simulink model "Simscape_exercise3"  (R2015b)
settings: Solver=ode23t  SolverMode=SingleTasking  StartTime=0.0  StopTime=5  RelTol=1e-3
values from neighbouring files (symbols this model uses):
  Amplitude = 2    [Exercise_3.m]
  Freq = 2    [Exercise_3.m]
  Jm = 7.46/(1000*100^2)    (= 7.46e-07)    [Exercise_1.m]    (also in Exercise_3.m)
  Sine_wave = 1    [Exercise_3.m]
  voltage = 1    [Exercise_3.m]
libraries: fl_lib x10, nesl_utility x6, simulink x1, elec_lib x1
settings Model: Creator=diegogm  LastModifiedBy=sofianh
settings DataIOCC: SaveFormat=Array
settings OptimizationCC: BlockReduction=off  BooleanDataType=off
settings DebuggingCC: SaveWithParameterizedLinksMsg=none  UnderspecifiedInitializationDetection=Classic  MergeDetectMultiDrivingBlocksExec=none  SignalResolutionControl=TryResolveAllWithWarning
settings HardwareCC: ProdBitPerPointer=32  ProdLargestAtomicFloat=None  ProdIntDivRoundTo=Undefined  ProdEndianess=Unspecified  ProdWordSize=32  ProdHWDeviceType=32-bit Generic  TargetUnknown=on
settings GRTTargetCC: GeneratePreprocessorConditionals=Disable all
settings ConfigComp: CovModelRefEnable=Off  CovSFcnEnable=off

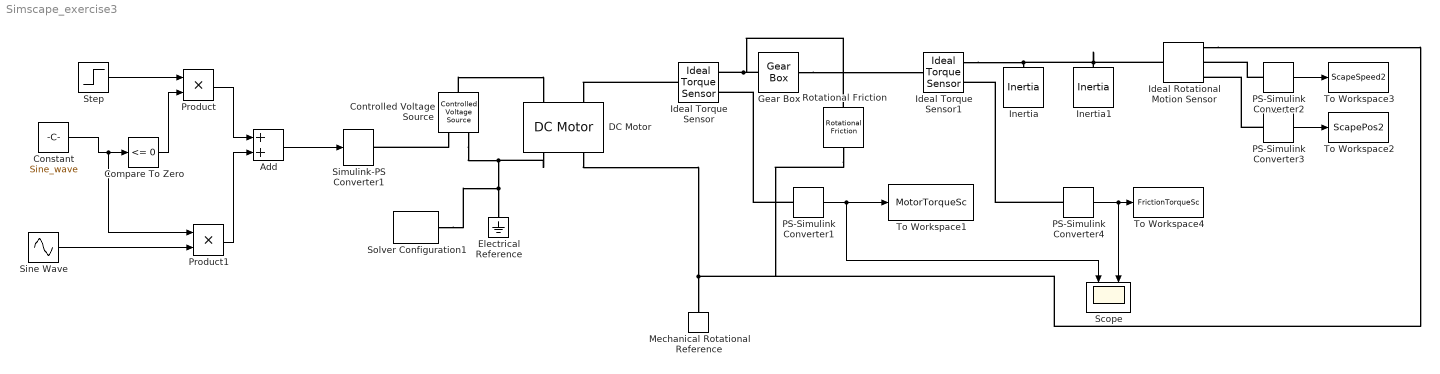
== system Simscape_exercise3 ==
  Add : Sum
  Compare To Zero : simulink/Logic and Bit Operations/Compare To Zero  relop=<=  OutDataTypeStr=boolean
  Constant : Constant  Value=Sine_wave
  Controlled Voltage Source : fl_lib/Electrical/Electrical Sources/Controlled Voltage Source
  DC Motor : elec_lib/Actuators & Drivers/Rotational Actuators/DC Motor  parameterization=1  Ra=R Ohm  La=L H  emf_or_torque=1  Kv=Kemf V/(rad/s)  Ki=6.876e-4 N*m/A  T_stall=2.4e-4 N*m  w_max=1.91e+4 rpm  w_rated=1.5e+4 rpm  P_rated=0.08 W  V_rated=1.5 V  J=Jm kg*m^2  lam_param=1  lam=dm N*m/(rad/s)  i_noload=0 A  V_i_noload=1.5 V  speed0=0 rpm  alpha=0.00393 1/K  Tmeas=25 C  thermal_mass=100 J/K  initial_temperature=25 C
  Electrical Reference : fl_lib/Electrical/Electrical Elements/Electrical Reference
  Gear Box : fl_lib/Mechanical/Mechanisms/Gear Box  ratio=n  t_in_specify=off  t_in_priority=High  t_in=0 N*m  t_out_specify=off  t_out_priority=High  t_out=0 N*m
  Ideal Rotational Motion Sensor : fl_lib/Mechanical/Mechanical Sensors/Ideal Rotational Motion Sensor  offset=0 rad
  Ideal Torque Sensor : fl_lib/Mechanical/Mechanical Sensors/Ideal Torque Sensor
  Ideal Torque Sensor1 : fl_lib/Mechanical/Mechanical Sensors/Ideal Torque Sensor
  Inertia : fl_lib/Mechanical/Rotational Elements/Inertia  inertia=J1 kg*m^2  w_specify=off  w_priority=High  w=0 rad/s  t_specify=off  t_priority=High  t=0 N*m
  Inertia1 : fl_lib/Mechanical/Rotational Elements/Inertia  inertia=J2 kg*m^2  w_specify=off  w_priority=High  w=0 rad/s  t_specify=off  t_priority=High  t=0 N*m
  Mechanical Rotational Reference : fl_lib/Mechanical/Rotational Elements/Mechanical Rotational Reference
  PS-Simulink Converter1 : nesl_utility/PS-Simulink Converter  PhysicalDomain=network_engine_domain  SubClassName=ps_output  LeftPortType=input  RightPortType=output  PseudoPeriodic=off  Frequencies=[]  Unit=N*m  AffineConversion=off
  PS-Simulink Converter2 : nesl_utility/PS-Simulink Converter  PhysicalDomain=network_engine_domain  SubClassName=ps_output  LeftPortType=input  RightPortType=output  PseudoPeriodic=off  Frequencies=[]  Unit=1  AffineConversion=off
  PS-Simulink Converter3 : nesl_utility/PS-Simulink Converter  PhysicalDomain=network_engine_domain  SubClassName=ps_output  LeftPortType=input  RightPortType=output  PseudoPeriodic=off  Frequencies=[]  Unit=1  AffineConversion=off
  PS-Simulink Converter4 : nesl_utility/PS-Simulink Converter  PhysicalDomain=network_engine_domain  SubClassName=ps_output  LeftPortType=input  RightPortType=output  PseudoPeriodic=off  Frequencies=[]  Unit=N*m  AffineConversion=off
  Product : Product
  Product1 : Product
  Rotational Friction : fl_lib/Mechanical/Rotational Elements/Rotational Friction  brkwy_trq=Tc N*m  Col_trq=Tc N*m  visc_coef=0 N*m/(rad/s)  trans_coef=1e-2 s/rad  vel_thr=1e-2 rad/s  w_specify=off  w_priority=None  w=0 rad/s  t_specify=off  t_priority=None  t=0 N*m
  Scope : Scope  NumInputPorts=2
  Simulink-PS Converter1 : nesl_utility/Simulink-PS Converter  PhysicalDomain=network_engine_domain  SubClassName=ps_input  LeftPortType=input  RightPortType=output  PseudoPeriodic=off  Frequencies=[]  NoiseDistribution=none  NoiseParameters=[]  Unit=1  AffineConversion=off  InputFiltering=off  SimscapeFilterOrder=1  InputFilterTimeConstant=0.001  UdotUserProvided=1
  Sine Wave : Sin  Amplitude=Amplitude  Frequency=Freq  SampleTime=0
  Solver Configuration1 : nesl_utility/Solver Configuration  PhysicalDomain=network_engine_domain  SubClassName=solver  LeftPortType=input  RightPortType=generic  Accelerate=off  Tones=[]  Harmonics=[]  SimulateNoise=off  Profile=off  UseLocalSampling=off  EnableSwitchedLinearOptims=on  FrequencyDomain=off  UseCCode=off  RelTol=0.001  AbsTol=1e-06  MinStep=1e-09  ToWorkspace=off  RevertToSquareIcSolve=off  NumHomotopyIterations=100  PhasorMode=off  PhasorModeNumHarmonics=1  DoDC=off  ResidualTolerance=1e-09  UseLocalSolver=off  LocalSolverChoice=NE_BACKWARD_EULER_ADVANCER  LocalSolverSampleTime=0.001  DoFixedCost=off  MaxNonlinIter=3  MaxModeIter=2  LinearAlgebra=Sparse  DelaysMemoryBudget=1024  AutomaticFiltering=on  FilteringTimeConstant=0.001
  Step : Step  Time=0  After=voltage  SampleTime=0
  To Workspace1 : ToWorkspace  VariableName=MotorTorqueSc  SaveFormat=Structure With Time  SampleTime=-1
  To Workspace2 : ToWorkspace  VariableName=ScapePos2  SaveFormat=Structure With Time  SampleTime=-1
  To Workspace3 : ToWorkspace  VariableName=ScapeSpeed2  SaveFormat=Structure With Time  SampleTime=-1
  To Workspace4 : ToWorkspace  VariableName=FrictionTorqueSc  SaveFormat=Structure With Time  SampleTime=-1
  wires:
  PS-Simulink Converter2/1 -> To Workspace3/1
  PS-Simulink Converter3/1 -> To Workspace2/1
  Add/1 -> Simulink-PS Converter1/1
  PS-Simulink Converter1/1 -> To Workspace1/1, Scope/1
  PS-Simulink Converter4/1 -> Scope/2, To Workspace4/1
  Step/1 -> Product/1
  Constant/1 -> Product1/1, Compare To Zero/1
  Sine Wave/1 -> Product1/2
  Product/1 -> Add/1
  Product1/1 -> Add/2
  Compare To Zero/1 -> Product/2
  connections:
  DC Motor/RConn1 -- Controlled Voltage Source/RConn2 -- Solver Configuration1/RConn1 -- Electrical Reference/LConn1
  DC Motor/RConn2 -- Rotational Friction/RConn1 -- Ideal Rotational Motion Sensor/RConn1 -- Mechanical Rotational Reference/LConn1
  Ideal Rotational Motion Sensor/LConn1 -- Inertia1/LConn1 -- Ideal Torque Sensor1/RConn1 -- Inertia/LConn1
  PS-Simulink Converter2/LConn1 -- Ideal Rotational Motion Sensor/RConn2
  PS-Simulink Converter3/LConn1 -- Ideal Rotational Motion Sensor/RConn3
  Controlled Voltage Source/RConn1 -- Simulink-PS Converter1/RConn1
  Controlled Voltage Source/LConn1 -- DC Motor/LConn1
  PS-Simulink Converter1/LConn1 -- Ideal Torque Sensor/RConn2
  PS-Simulink Converter4/LConn1 -- Ideal Torque Sensor1/RConn2
  Gear Box/RConn1 -- Ideal Torque Sensor1/LConn1
  Gear Box/LConn1 -- Ideal Torque Sensor/RConn1 -- Rotational Friction/LConn1
  Ideal Torque Sensor/LConn1 -- DC Motor/LConn2
